simulink model "power_3phseriescomp"  (R2022a)
settings: Solver=FixedStepDiscrete  StartTime=0.0  StopTime=0.2  FixedStep=Ts  RelTol=1e-4  EnableMultiTasking=on
PreLoadFcn:
  | Ts=50e-6;
InitFcn:
  | Ts=50e-6;
undefined symbols (not defined in the file): D1, Delta, DiscIntNeverNeededParam
libraries: spsSeriesRLCBranchLib x6, spsBreakerLib x6, spsCurrentMeasurementLib x6, spsSurgeArresterLib x6, spsParallelRLCBranchLib x6, spsVoltageMeasurementLib x6, spsThreePhaseSeriesRLCLoadLib x4, spsLoadFlowBusLib x4, spsThreePhaseVIMeasurementLib x3, spsThreePhaseBreakerLib x2, spsDistributedParametersLineLib x2, spsThreePhaseSourceLib x1
(part 2 of 2)

== system power_3phseriescomp/Series Compensation (unit 2) /Phase A2/Energy & Gap firing ==
  note: Latch
  I_MOV : Inport
  U_MOV : Inport  Port=2
  Discrete-Time Integrator : DiscreteIntegrator  SampleTime=Ts  ICPrevOutput=DiscIntNeverNeededParam  ICPrevScaledInput=DiscIntNeverNeededParam
  MOV Energy Threshold : Constant  Value=30e6
  Product : Product  InputSameDT=on  SaturateOnIntegerOverflow=on  OutDataTypeStr=Inherit: Same as first input
  Relational Operator : RelationalOperator  Operator=>  ZeroCross=off
  Switch : Switch  Threshold=0.5  ZeroCross=off  SaturateOnIntegerOverflow=off
  Unit Delay : UnitDelay  SampleTime=Ts  HasFrameUpgradeWarning=on
  Gap_trip : Outport  VectorParamsAs1DForOutWhenUnconnected=off
  wires:
  Unit Delay/1 -> Switch/3
  Relational Operator/1 -> Switch/2, Switch/1
  Discrete-Time Integrator/1 -> Relational Operator/1
  I_MOV/1 -> Product/1
  Product/1 -> Discrete-Time Integrator/1
  MOV Energy Threshold/1 -> Relational Operator/2
  U_MOV/1 -> Product/2
  Switch/1 -> Gap_trip/1, Unit Delay/1
